simulink model "mass_and_grad_est"  (R2024a)
settings: Solver=ode4  StartTime=0.0  StopTime=300  FixedStep=0.001  RelTol=1e-3
undefined symbols (not defined in the file): filt_damp
settings Model: Creator=sriva  LastModifiedBy=sriva
settings OptimizationCC: ReuseModelBlockBuffer=off
settings RTWCC: GPUComputeCapability=3.5

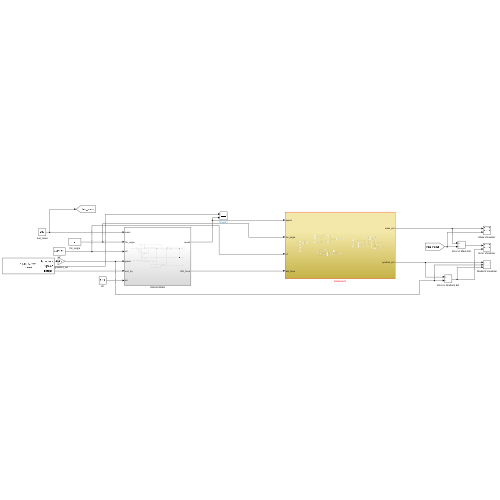
[thumbnail: Simulink's stored preview of the top-level diagram]
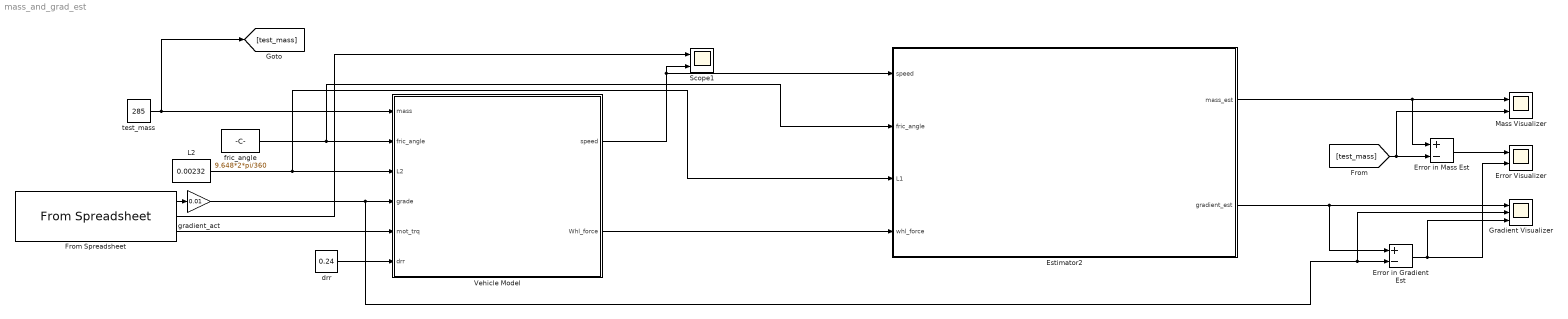
== system mass_and_grad_est ==
  Error Visualizer : Scope  NumInputPorts=2
  Error in Gradient Est : Sum  Inputs=+-
  Error in Mass Est : Sum  Inputs=+-
  Estimator2 : Subsystem
  From Spreadsheet : FromSpreadsheet  FileName=grade_def.xlsx
  Gradient Visualizer : Scope  NumInputPorts=3
  L2 : Constant  Value=0.00232
  Mass Visualizer : Scope  NumInputPorts=2
  Scope1 : Scope  NumInputPorts=2
  Vehicle Model : Subsystem
  drr : Constant  Value=0.24
  fric_angle : Constant  Value=9.648*2*pi/360
  gradient_act : Gain  Gain=0.01
  test_mass : Constant  Value=285
  wires:
  fric_angle/1 -> Estimator2/2(fric_angle), Vehicle Model/2(fric_angle)
  L2/1 -> Estimator2/3(L1), Vehicle Model/3(L2)
  Vehicle Model/1(speed) -> Scope1/2, Estimator2/1(speed)
  test_mass/1 -> [test_mass], Vehicle Model/1(mass)
  From Spreadsheet/3 -> Vehicle Model/5(mot_trq)
  drr/1 -> Vehicle Model/6(drr)
  From Spreadsheet/1 -> gradient_act/1
  Vehicle Model/2(Whl_force) -> Estimator2/4(whl_force)
  Estimator2/2(gradient_est) -> Error in Gradient Est/1, Gradient Visualizer/1
  From Spreadsheet/2 -> Scope1/1
  Estimator2/1(mass_est) -> Error in Mass Est/1, Mass Visualizer/1
  gradient_act/1 -> Error in Gradient Est/2, Gradient Visualizer/2, Vehicle Model/4(grade)
  Error in Gradient Est/1 -> Gradient Visualizer/3, Error Visualizer/2
  [test_mass] -> Mass Visualizer/2, Error in Mass Est/2
  Error in Mass Est/1 -> Error Visualizer/1

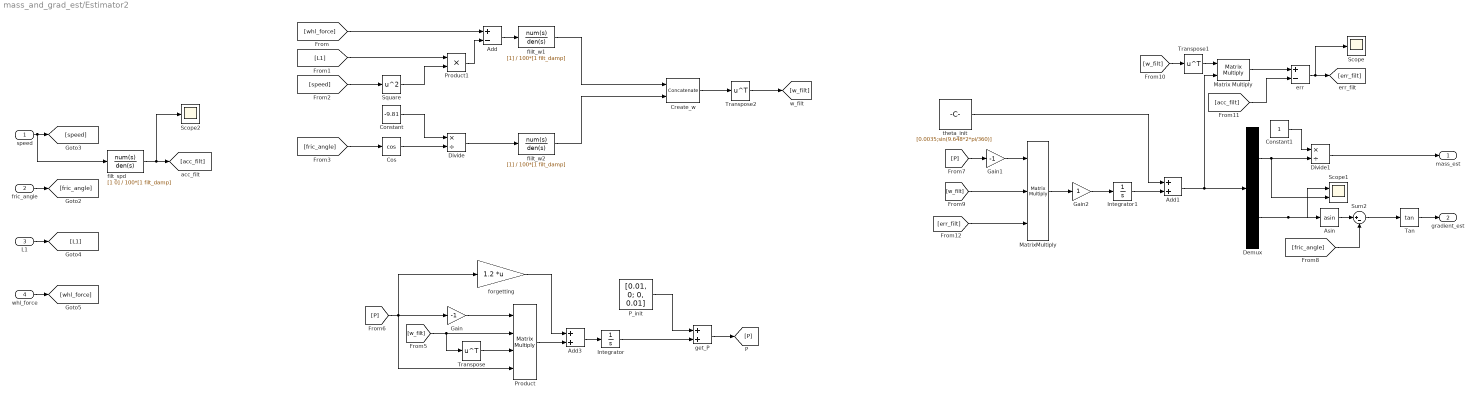
== system mass_and_grad_est/Estimator2 ==
  speed : Inport
  fric_angle : Inport  Port=2
  L1 : Inport  Port=3
  whl_force : Inport  Port=4
  Add : Sum  Inputs=+-
  Add1 : Sum
  Add3 : Sum
  Asin : Trigonometry  Operator=asin
  Constant : Constant  Value=-9.81
  Constant1 : Constant
  Cos : Trigonometry  Operator=cos
  Create_w : Concatenate  Mode=Multidimensional array  ConcatenateDimension=2
  Demux : Demux  Outputs=2
  Divide : Product  Inputs=*/
  Divide1 : Product  Inputs=*/
  Gain : Gain  Gain=-1
  Gain1 : Gain  Gain=-1
  Gain2 : Gain
  Integrator : Integrator
  Integrator1 : Integrator
  Matrix Multiply : Product  Multiplication=Matrix(*)
  MatrixMultiply : Product  Inputs=3  Multiplication=Matrix(*)
  P_init : Constant  Value=[0.01, 0; 0, 0.01]
  Product : Product  Inputs=4  Multiplication=Matrix(*)
  Product1 : Product
  Scope : Scope
  Scope1 : Scope  NumInputPorts=2
  Scope2 : Scope
  Square : Math  Operator=square
  Sum2 : Sum  Inputs=|+-
  Tan : Trigonometry  Operator=tan
  Transpose : Math  Operator=transpose
  Transpose1 : Math  Operator=transpose
  Transpose2 : Math  Operator=transpose
  err : Sum  Inputs=+-
  filt_spd : TransferFcn  Numerator=[1 0]  Denominator=100*[1 filt_damp]
  flilt_w1 : TransferFcn  Denominator=100*[1 filt_damp]
  flilt_w2 : TransferFcn  Denominator=100*[1 filt_damp]
  forgetting : Gain  Gain=1.2  Multiplication=Matrix(K*u)
  get_P : Sum
  theta_init : Constant  Value=[0.0035;sin(9.648*2*pi/360)]  VectorParams1D=off
  mass_est : Outport
  gradient_est : Outport  Port=2
  wires:
  L1/1 -> [L1]
  fric_angle/1 -> [fric_angle]
  whl_force/1 -> [whl_force]
  [speed] -> Square/1
  Square/1 -> Product1/2
  [L1] -> Product1/1
  [whl_force] -> Add/1
  Product1/1 -> Add/2
  [fric_angle] -> Cos/1
  Constant/1 -> Divide/1
  Cos/1 -> Divide/2
  Add/1 -> flilt_w1/1
  Divide/1 -> flilt_w2/1
  speed/1 -> filt_spd/1, [speed]
  flilt_w2/1 -> Create_w/2
  flilt_w1/1 -> Create_w/1
  Asin/1 -> Sum2/1
  Tan/1 -> gradient_est/1
  Sum2/1 -> Tan/1
  Add1/1 -> Matrix Multiply/2, Demux/1
  [fric_angle] -> Sum2/2
  Divide1/1 -> mass_est/1
  Demux/2 -> Scope1/1, Asin/1
  P_init/1 -> get_P/1
  Create_w/1 -> Transpose2/1
  [w_filt] -> Transpose/1, Product/2
  Transpose/1 -> Product/3
  [P] -> forgetting/1, Product/4, Gain/1
  Integrator/1 -> get_P/2
  Gain/1 -> Product/1
  get_P/1 -> [P]
  [P] -> Gain1/1
  Gain1/1 -> MatrixMultiply/1
  [w_filt] -> MatrixMultiply/2
  MatrixMultiply/1 -> Gain2/1
  Integrator1/1 -> Add1/2
  theta_init/1 -> Add1/1
  [w_filt] -> Transpose1/1
  Transpose1/1 -> Matrix Multiply/1
  filt_spd/1 -> Scope2/1, [acc_filt]
  [acc_filt] -> err/2
  Matrix Multiply/1 -> err/1
  err/1 -> Scope/1, [err_filt]
  [err_filt] -> MatrixMultiply/3
  Transpose2/1 -> [w_filt]
  Product/1 -> Add3/2
  forgetting/1 -> Add3/1
  Add3/1 -> Integrator/1
  Gain2/1 -> Integrator1/1
  Demux/1 -> Scope1/2, Divide1/2
  Constant1/1 -> Divide1/1

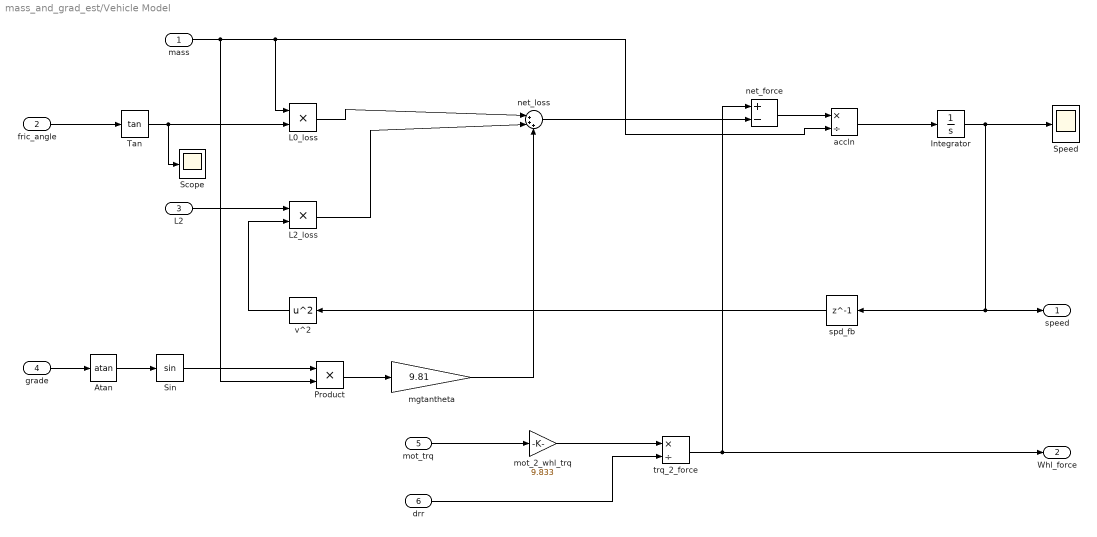
== system mass_and_grad_est/Vehicle Model ==
  mass : Inport
  fric_angle : Inport  Port=2
  L2 : Inport  Port=3
  grade : Inport  Port=4
  mot_trq : Inport  Port=5
  drr : Inport  Port=6
  Atan : Trigonometry  Operator=atan
  Integrator : Integrator
  L0_loss : Product
  L2_loss : Product
  Product : Product
  Scope : Scope
  Sin : Trigonometry
  Speed : Scope
  Tan : Trigonometry  Operator=tan
  accln : Product  Inputs=*/
  mgtantheta : Gain  Gain=9.81
  mot_2_whl_trq : Gain  Gain=9.833
  net_force : Sum  Inputs=+-
  net_loss : Sum  Inputs=|+++
  spd_fb : Delay  DelayLength=1  InitialCondition=0
  trq_2_force : Product  Inputs=*/
  v^2 : Math  Operator=square
  speed : Outport
  Whl_force : Outport  Port=2
  wires:
  mot_trq/1 -> mot_2_whl_trq/1
  mass/1 -> accln/2, L0_loss/1, Product/2
  L2/1 -> L2_loss/1
  L0_loss/1 -> net_loss/1
  L2_loss/1 -> net_loss/2
  mot_2_whl_trq/1 -> trq_2_force/1
  drr/1 -> trq_2_force/2
  trq_2_force/1 -> Whl_force/1, net_force/1
  net_loss/1 -> net_force/2
  v^2/1 -> L2_loss/2
  spd_fb/1 -> v^2/1
  net_force/1 -> accln/1
  accln/1 -> Integrator/1
  Integrator/1 -> Speed/1, speed/1, spd_fb/1
  grade/1 -> Atan/1
  Product/1 -> mgtantheta/1
  mgtantheta/1 -> net_loss/3
  fric_angle/1 -> Tan/1
  Tan/1 -> Scope/1, L0_loss/2
  Atan/1 -> Sin/1
  Sin/1 -> Product/1
